simulink model "FINAL_CSD_9LEVEL_SPWM_FIXED_DC_2"  (R2014a)
settings: Solver=ode45  StartTime=0.02  StopTime=0.4  RelTol=1e-3
libraries: powerlib x30, simulink x8
settings Model: Creator=PRAKASH BABU  LastModifiedBy=PRAKASH BABU

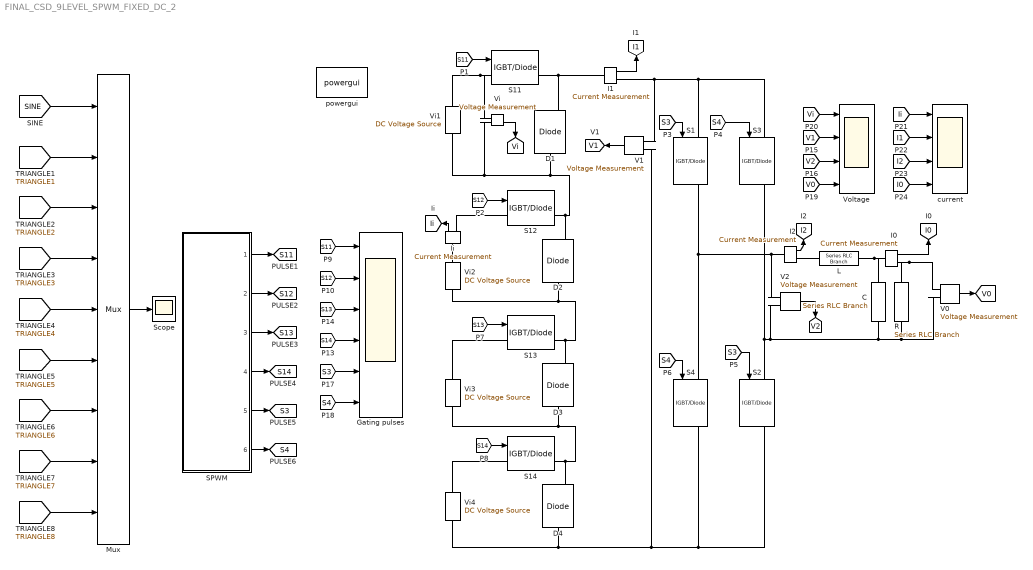
== system FINAL_CSD_9LEVEL_SPWM_FIXED_DC_2 ==
  C : powerlib/Elements/Series RLC Branch  LConnTagsString=__new0  RConnTagsString=__new0  BranchType=C  Resistance=1  Inductance=0.1  SetiL0=off  InitialCurrent=0  Capacitance=7e-6  Setx0=off  InitialVoltage=0  Measurements=None
  D{1..4} (4 alike) : powerlib/Power Electronics/Diode  Ron=0.001  Lon=0  Vf=0.8  IC=0  UseSnubber=off  Rs=500  Cs=250e-9  Measurements=on
  Gating pulses : Scope  NumInputPorts=6
      settings: YMin=-5~-5~-5~-5~-5~-5  YMax=5~5~5~5~5~5  SaveName=gate
  I0 : powerlib/Measurements/Current Measurement  PhasorSimulation=off  OutputType=Complex  PSBequivalent=0
  I1 : powerlib/Measurements/Current Measurement  PhasorSimulation=off  OutputType=Complex  PSBequivalent=0
  I2 : powerlib/Measurements/Current Measurement  PhasorSimulation=off  OutputType=Complex  PSBequivalent=0
  Ii : powerlib/Measurements/Current Measurement  PhasorSimulation=off  OutputType=Complex  PSBequivalent=0
  L : powerlib/Elements/Series RLC Branch  LConnTagsString=__new0  RConnTagsString=__new0  BranchType=L  Resistance=1  Inductance=61e-3  SetiL0=off  InitialCurrent=0  Capacitance=1e-6  Setx0=off  InitialVoltage=0  Measurements=None
  Mux : Mux  Inputs=9
  R : powerlib/Elements/Series RLC Branch  LConnTagsString=__new0  RConnTagsString=__new0  BranchType=R  Resistance=90  Inductance=20e-6  SetiL0=off  InitialCurrent=0  Capacitance=1e-6  Setx0=off  InitialVoltage=0  Measurements=None
  S{1..4,11..14} (8 alike) : powerlib/Power Electronics/IGBT//Diode  Ron=1e-3  Rs=1e5  Cs=inf  Measurements=on
  SPWM : Subsystem
  Scope : Scope
      settings: TickLabels=on  SaveName=sine
  V0 : powerlib/Measurements/Voltage Measurement  PhasorSimulation=off  OutputType=Complex  PSBequivalent=0
  V1 : powerlib/Measurements/Voltage Measurement  PhasorSimulation=off  OutputType=Complex  PSBequivalent=0
  V2 : powerlib/Measurements/Voltage Measurement  PhasorSimulation=off  OutputType=Complex  PSBequivalent=0
  Vi : powerlib/Measurements/Voltage Measurement  PhasorSimulation=off  OutputType=Complex  PSBequivalent=0
  Vi1 : powerlib/Electrical Sources/DC Voltage Source  Amplitude=57.5  Measurements=None
  Vi2 : powerlib/Electrical Sources/DC Voltage Source  Amplitude=57.5  Measurements=None
  Vi3 : powerlib/Electrical Sources/DC Voltage Source  Amplitude=57.5  Measurements=None
  Vi4 : powerlib/Electrical Sources/DC Voltage Source  Amplitude=57.4  Measurements=None
  Voltage : Scope  NumInputPorts=4
      settings: TimeRange=0.08  YMin=57.25~0~-400~-400  YMax=57.5~250~400~400  SaveName=voltage
  current : Scope  NumInputPorts=4
      settings: YMin=0~-5~-230~-5  YMax=70~5~230~5  SaveName=current
  powergui : powerlib/powergui  Priority=1  SimulationMode=Discrete  SolverType=Tustin  SampleTime=50e-6  frequency=60  SPID=off  DisableSnubberDevices=off  DisableRonSwitches=off  DisableVfSwitches=off  SwTol=0  Interpol=off  DisplayEquations=off  Ts=0  methode=off  frequencyindice=0  Pbase=100e6  ErrMax=1e-4  Iterations=50  UnitsV=kV  UnitsW=MW  FunctionMessages=off  echomessages=off  HookPort=off  EnableUseOfTLC=off  x0status=blocks  RestoreLinks=warning  ResistiveCurrentMeasurement=off  Frange=[0:2:500]  Ylog=off  Xlog=on  ShowGrid=off  save=off  variable=ZData  structure=Voltage1  ZoomFFT=off  StartTime=0.04  cycles=1  DisplayStyle=1  fundamental=50  FreqAxis=off  MaxFrequency=1000  frequencyindicesteady=1  RmsSteady=1  display=off
  tag scope: I0=global, I1=global, I2=global, Ii=global, S11=global, S12=global, S13=global, S14=global, S3=global, S4=global, V0=global, V1=global, V2=global, Vi=global
  wires:
  V0/1 -> [V0]
  [S11] -> S11/1
  [S12] -> S12/1
  [S4] -> S3/1
  [S3] -> S1/1
  [S4] -> S4/1
  [S3] -> S2/1
  [S14] -> S14/1
  [S13] -> S13/1
  [SINE] -> Mux/1
  [TRIANGLE1] -> Mux/2
  [TRIANGLE2] -> Mux/3
  [TRIANGLE3] -> Mux/4
  [TRIANGLE4] -> Mux/5
  Mux/1 -> Scope/1
  [S12] -> Gating pulses/2
  [S13] -> Gating pulses/3
  [S14] -> Gating pulses/4
  [TRIANGLE5] -> Mux/6
  [TRIANGLE6] -> Mux/7
  [TRIANGLE7] -> Mux/8
  [TRIANGLE8] -> Mux/9
  [S3] -> Gating pulses/5
  [S4] -> Gating pulses/6
  SPWM/1(1) -> [S11]
  SPWM/2(2) -> [S12]
  SPWM/3(3) -> [S13]
  SPWM/4(4) -> [S14]
  [S11] -> Gating pulses/1
  SPWM/6(6) -> [S4]
  SPWM/5(5) -> [S3]
  V1/1 -> [V1]
  V2/1 -> [V2]
  Vi/1 -> [Vi]
  [V1] -> Voltage/2
  [V2] -> Voltage/3
  [V0] -> Voltage/4
  [Vi] -> Voltage/1
  [I0] -> current/4
  [I2] -> current/3
  [I1] -> current/2
  [Ii] -> current/1
  Ii/1 -> [Ii]
  I1/1 -> [I1]
  I2/1 -> [I2]
  I0/1 -> [I0]
  connections:
  D4/LConn1 -- Vi4/LConn1 -- S4/RConn1 -- S2/RConn1 -- V1/LConn2
  V0/LConn2 -- R/RConn1 -- V2/LConn2 -- S3/RConn1 -- S2/LConn1 -- C/RConn1
  V1/LConn1 -- I1/RConn1 -- S3/LConn1 -- S1/LConn1
  D1/LConn1 -- Vi/LConn2 -- Vi1/LConn1 -- D2/RConn1 -- S12/RConn1
  S14/RConn1 -- Vi3/LConn1 -- D3/LConn1 -- D4/RConn1
  S13/LConn1 -- Vi3/RConn1
  S14/LConn1 -- Vi4/RConn1
  D3/RConn1 -- Vi2/LConn1 -- D2/LConn1 -- S13/RConn1
  S1/RConn1 -- S4/LConn1 -- V2/LConn1 -- I2/LConn1
  C/LConn1 -- I0/LConn1 -- L/LConn1
  S11/LConn1 -- Vi1/RConn1 -- Vi/LConn1
  Vi2/RConn1 -- Ii/LConn1
  Ii/RConn1 -- S12/LConn1
  S11/RConn1 -- I1/LConn1 -- D1/RConn1
  I2/RConn1 -- L/RConn1
  R/LConn1 -- I0/RConn1 -- V0/LConn1

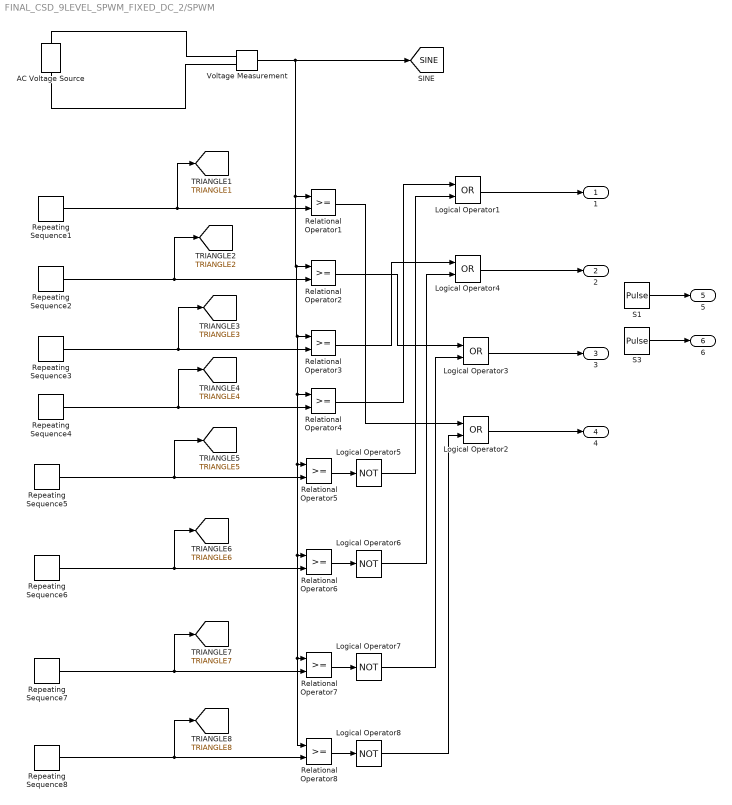
== system FINAL_CSD_9LEVEL_SPWM_FIXED_DC_2/SPWM ==
  AC Voltage Source : powerlib/Electrical Sources/AC Voltage Source  Amplitude=4  Phase=0  Frequency=50  SampleTime=0  Measurements=None
  Logical Operator{1..4} (4 alike) : Logic  Operator=OR  AllPortsSameDT=off  OutDataTypeStr=boolean
  Logical Operator{5..8} (4 alike) : Logic  Operator=NOT  AllPortsSameDT=off  OutDataTypeStr=boolean
  Relational Operator{1..8} (8 alike) : RelationalOperator  OutDataTypeStr=boolean
  Repeating Sequence1 : simulink/Sources/Repeating Sequence  rep_seq_t=[0 0.5 1]/2500  rep_seq_y=[3 4 3]
  Repeating Sequence2 : simulink/Sources/Repeating Sequence  rep_seq_t=[0 0.5 1]/2500  rep_seq_y=[2 3 2]
  Repeating Sequence3 : simulink/Sources/Repeating Sequence  rep_seq_t=[0 0.5 1]/2500  rep_seq_y=[1 2 1]
  Repeating Sequence4 : simulink/Sources/Repeating Sequence  rep_seq_t=[0 0.5 1]/2500  rep_seq_y=[0 1 0]
  Repeating Sequence5 : simulink/Sources/Repeating Sequence  rep_seq_t=[0 0.5 1]/2500  rep_seq_y=[-1 0 -1]
  Repeating Sequence6 : simulink/Sources/Repeating Sequence  rep_seq_t=[0 0.5 1]/2500  rep_seq_y=[-2 -1 -2]
  Repeating Sequence7 : simulink/Sources/Repeating Sequence  rep_seq_t=[0 0.5 1]/2500  rep_seq_y=[-3 -2 -3]
  Repeating Sequence8 : simulink/Sources/Repeating Sequence  rep_seq_t=[0 0.5 1]/2500  rep_seq_y=[-4 -3 -4]
  S1 : DiscretePulseGenerator  PulseType=Time based  Period=0.02  PulseWidth=50
  S3 : DiscretePulseGenerator  PulseType=Time based  Period=0.02  PulseWidth=50  PhaseDelay=0.01
  Voltage Measurement : powerlib/Measurements/Voltage Measurement  PhasorSimulation=off  OutputType=Complex  PSBequivalent=0
  1 : Outport
  2 : Outport  Port=2
  3 : Outport  Port=3
  4 : Outport  Port=4
  5 : Outport  Port=5
  6 : Outport  Port=6
  tag scope: SINE=global, TRIANGLE1=global, TRIANGLE2=global, TRIANGLE3=global, TRIANGLE4=global, TRIANGLE5=global, TRIANGLE6=global, TRIANGLE7=global, TRIANGLE8=global
  wires:
  Repeating Sequence2/1 -> [TRIANGLE2], Relational Operator2/2
  Voltage Measurement/1 -> Relational Operator4/1, Relational Operator6/1, Relational Operator7/1, Relational Operator8/1, Relational Operator5/1, Relational Operator3/1, Relational Operator2/1, Relational Operator1/1, [SINE]
  Repeating Sequence1/1 -> [TRIANGLE1], Relational Operator1/2
  Repeating Sequence3/1 -> [TRIANGLE3], Relational Operator3/2
  Repeating Sequence4/1 -> [TRIANGLE4], Relational Operator4/2
  Repeating Sequence5/1 -> [TRIANGLE5], Relational Operator5/2
  Logical Operator5/1 -> Logical Operator1/2
  Relational Operator6/1 -> Logical Operator6/1
  Repeating Sequence6/1 -> [TRIANGLE6], Relational Operator6/2
  Logical Operator6/1 -> Logical Operator4/2
  Relational Operator7/1 -> Logical Operator7/1
  Repeating Sequence7/1 -> [TRIANGLE7], Relational Operator7/2
  Logical Operator7/1 -> Logical Operator3/2
  Relational Operator8/1 -> Logical Operator8/1
  Repeating Sequence8/1 -> [TRIANGLE8], Relational Operator8/2
  Logical Operator8/1 -> Logical Operator2/2
  Relational Operator5/1 -> Logical Operator5/1
  Relational Operator4/1 -> Logical Operator1/1
  Relational Operator3/1 -> Logical Operator4/1
  Relational Operator2/1 -> Logical Operator3/1
  Relational Operator1/1 -> Logical Operator2/1
  Logical Operator1/1 -> 1/1
  Logical Operator3/1 -> 3/1
  Logical Operator2/1 -> 4/1
  S1/1 -> 5/1
  S3/1 -> 6/1
  Logical Operator4/1 -> 2/1
  connections:
  AC Voltage Source/LConn1 -- Voltage Measurement/LConn2
  AC Voltage Source/RConn1 -- Voltage Measurement/LConn1
